simulink model "Caracterizacionprueba"  (R2022b)
settings: Solver=VariableStepAuto  StartTime=0.0  StopTime=inf  RelTol=1e-3
libraries: robotlib x3
settings Model: Creator=alanraven60  LastModifiedBy=alex

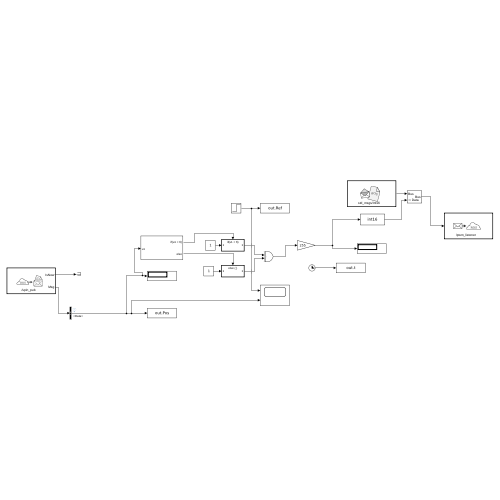
[thumbnail: Simulink's stored preview of the top-level diagram]
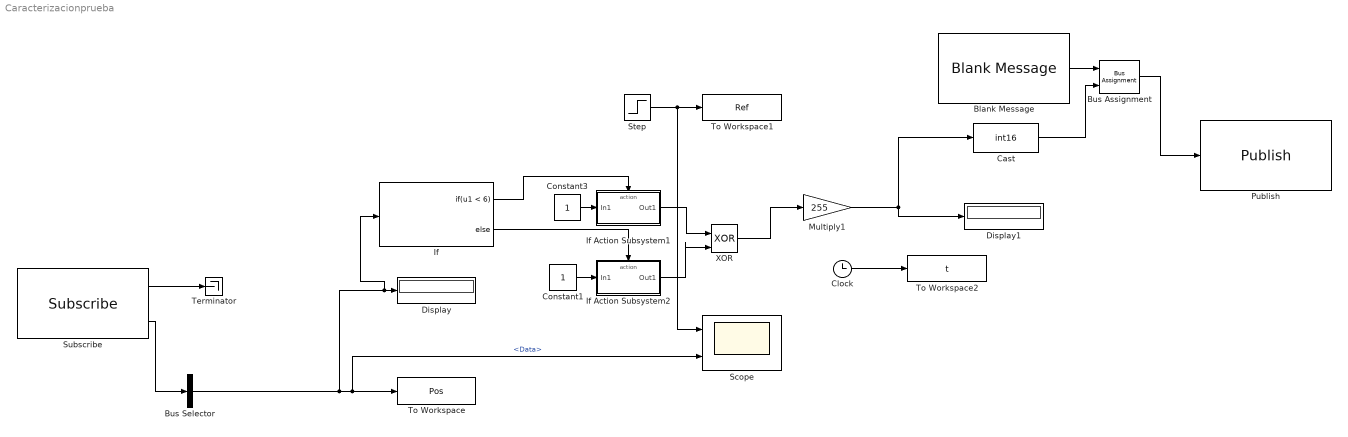
== system Caracterizacionprueba ==
  Blank Message : robotlib/Blank Message  messageClass=Message  entityType=std_msgs/Int16  messageType=std_msgs/Int16  SampleTime=inf  legacyBusStruct=off
      settings: LibrarySourceBlock=roslib/ROS/Blank Message
  Bus Assignment : BusAssignment  AssignedSignals=Data
  Bus Selector : BusSelector  OutputSignals=Data
  Cast : DataTypeConversion  OutDataTypeStr=int16  SaturateOnIntegerOverflow=off  RndMeth=Floor
  Clock : Clock
  Constant1 : Constant
  Constant3 : Constant
  Display : Display
  Display1 : Display
  If : If  IfExpression=u1 < 6  ZeroCross=off
  If Action Subsystem1 : Subsystem  TreatAsAtomicUnit=on
  If Action Subsystem2 : Subsystem  TreatAsAtomicUnit=on
  Multiply1 : Gain  Gain=255
  Publish : robotlib/Publish  topicSource=Select from ROS network  topic=/pwm_listener  messageType=std_msgs/Int16  legacyBusStruct=off  messageQueueLength=1
      settings: LibrarySourceBlock=roslib/ROS/Publish
  Scope : Scope  NumInputPorts=2
  Step : Step  Time=0  After=6.446  SampleTime=0
  Subscribe : robotlib/Subscribe  topicSource=Select from ROS network  topic=/spin_pub  messageType=std_msgs/Float32  SampleTime=-1  legacyBusStruct=off  messageQueueLength=1
      settings: LibrarySourceBlock=roslib/ROS/Subscribe
  Terminator : Terminator
  To Workspace : ToWorkspace  VariableName=Pos  SaveFormat=Timeseries  SampleTime=0.01
  To Workspace1 : ToWorkspace  VariableName=Ref  SaveFormat=Timeseries  SampleTime=0.01
  To Workspace2 : ToWorkspace  VariableName=t  SaveFormat=Timeseries  SampleTime=0.01
  XOR : Logic  Operator=XOR  IconShape=distinctive  AllPortsSameDT=off  OutDataTypeStr=boolean
  wires:
  Subscribe/1 -> Terminator/1
  Subscribe/2 -> Bus Selector/1
  Clock/1 -> To Workspace2/1
  Blank Message/1 -> Bus Assignment/1
  Bus Assignment/1 -> Publish/1
  Cast/1 -> Bus Assignment/2
  Bus Selector/1 -> Scope/2, To Workspace/1, If/1, Display/1  "<Data>"
  If Action Subsystem1/1(Out1) -> XOR/1
  Constant3/1 -> If Action Subsystem1/1(In1)
  If/1 -> If Action Subsystem1/Action
  XOR/1 -> Multiply1/1
  Step/1 -> Scope/1, To Workspace1/1
  Multiply1/1 -> Display1/1, Cast/1
  If/2 -> If Action Subsystem2/Action
  Constant1/1 -> If Action Subsystem2/1(In1)
  If Action Subsystem2/1(Out1) -> XOR/2

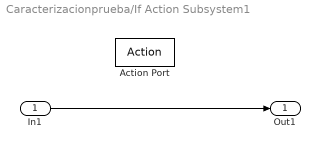
== system Caracterizacionprueba/If Action Subsystem1 ==
  In1 : Inport
  Action Port : ActionPort  ActionPortLabel=if(u1 < 6)
  Out1 : Outport
  wires:
  In1/1 -> Out1/1

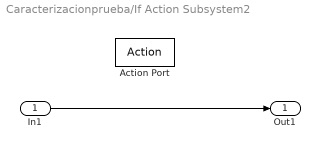
== system Caracterizacionprueba/If Action Subsystem2 ==
  In1 : Inport
  Action Port : ActionPort  ActionPortLabel=else
  Out1 : Outport
  wires:
  In1/1 -> Out1/1
